simulink model "LLC_simscape3"  (R2022b)
settings: Solver=VariableStepAuto  StartTime=0.0  StopTime=0.1  MaxStep=1e-4  RelTol=1e-4
PreLoadFcn:
  | Rs_fet=1e8;  % FET snubber resistance (ohms)
  | Cs_fet=inf;  % FET snubber capacitance (ohms)
  | Vf=0.6;        % Diode forward voltage (V)
libraries: spsSeriesRLCBranchLib x10, spsVoltageMeasurementLib x7, spsCurrentMeasurementLib x5, spsControlledVoltageSourceLib x2, spsGroundLib x2, spsNonlinearInductorLib x2, spsACVoltageSourceLib x1, spspowerguiLib x1
settings Model: SimulationMode=accelerator  PauseTimes=0.001  Creator=Hyeongmeen Baik  LastModifiedBy=Hyeongmeen Baik
settings ModelReferenceCC: UpdateModelReferenceTargets=IfOutOfDate  EnableRefExpFcnMdlSchedulingChecks=on

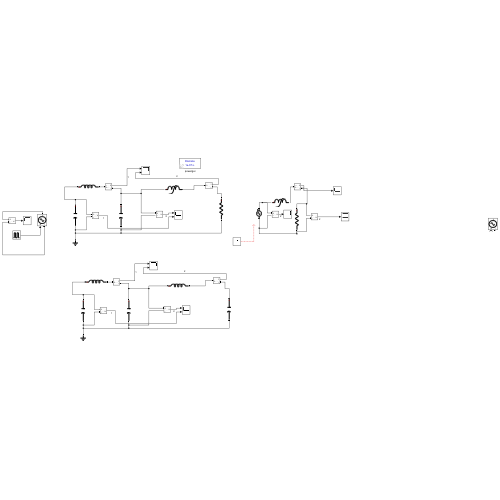
[thumbnail: Simulink's stored preview of the top-level diagram]
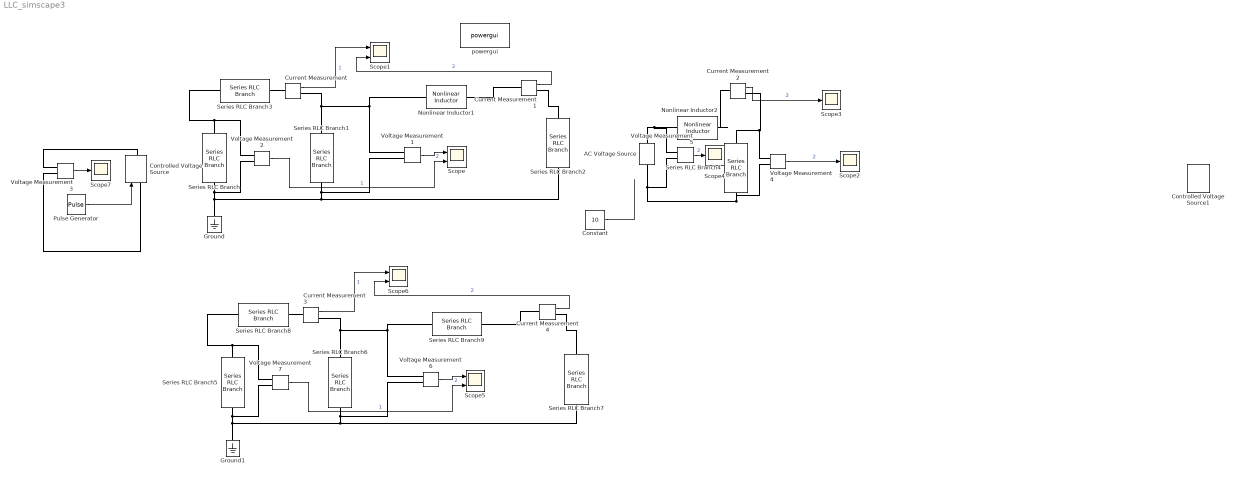
== system LLC_simscape3 ==
  AC Voltage Source : spsACVoltageSourceLib/AC Voltage Source  Amplitude=1500  Phase=0  Frequency=10  SampleTime=0  Measurements=None  BusType=swing  Pref=10e3  Qref=0  Qmin=-inf  Qmax=+inf
  Constant : Constant  Value=10
  Controlled Voltage Source : spsControlledVoltageSourceLib/Controlled Voltage Source  Initialize=on  Source_Type=AC  Amplitude=0  Phase=0  Frequency=0  Measurements=None
  Controlled Voltage Source1 : spsControlledVoltageSourceLib/Controlled Voltage Source  Initialize=on  Source_Type=AC  Amplitude=0  Phase=0  Frequency=0  Measurements=None
  Current Measurement{,1..4} (5 alike) : spsCurrentMeasurementLib/Current Measurement  PhasorSimulation=off  OutputType=Complex  PSBequivalent=0
  Ground : spsGroundLib/Ground  LConnTagsString=a
  Ground1 : spsGroundLib/Ground  LConnTagsString=a
  Nonlinear Inductor1 : spsNonlinearInductorLib/Nonlinear Inductor  DiscreteSolver=Backward Euler  VI=flux_current2  IFL=0  Measurements=Flux, Imag
      settings: LibrarySourceBlock=sps_lib/Passives/Nonlinear Inductor
  Nonlinear Inductor2 : spsNonlinearInductorLib/Nonlinear Inductor  DiscreteSolver=Backward Euler  VI=flux_current2  IFL=0  Measurements=Flux, Imag
      settings: LibrarySourceBlock=sps_lib/Passives/Nonlinear Inductor
  Pulse Generator : DiscretePulseGenerator  PulseType=Time based  Period=0.1  PulseWidth=5
  Scope{,1,5..6} (4 alike) : Scope  NumInputPorts=2
  Scope{2..4,7} (4 alike) : Scope
  Series RLC Branch : spsSeriesRLCBranchLib/Series RLC Branch  LConnTagsString=__new0  RConnTagsString=__new0  BranchType=C  Resistance=1  Inductance=1e-3  SetiL0=off  InitialCurrent=0  Capacitance=1e-3  Setx0=on  InitialVoltage=1500  Measurements=None
  Series RLC Branch1 : spsSeriesRLCBranchLib/Series RLC Branch  LConnTagsString=__new0  RConnTagsString=__new0  BranchType=C  Resistance=1  Inductance=1e-3  SetiL0=off  InitialCurrent=0  Capacitance=1e-3  Setx0=off  InitialVoltage=0  Measurements=None
  Series RLC Branch2 : spsSeriesRLCBranchLib/Series RLC Branch  LConnTagsString=__new0  RConnTagsString=__new0  BranchType=R  Resistance=1  Inductance=1e-3  SetiL0=off  InitialCurrent=0  Capacitance=1e-6  Setx0=off  InitialVoltage=0  Measurements=None
  Series RLC Branch3 : spsSeriesRLCBranchLib/Series RLC Branch  LConnTagsString=__new0  RConnTagsString=__new0  BranchType=L  Resistance=1  Inductance=1e-3  SetiL0=off  InitialCurrent=0  Capacitance=1e-6  Setx0=off  InitialVoltage=0  Measurements=None
  Series RLC Branch4 : spsSeriesRLCBranchLib/Series RLC Branch  LConnTagsString=__new0  RConnTagsString=__new0  BranchType=R  Resistance=1  Inductance=1e-3  SetiL0=off  InitialCurrent=0  Capacitance=1e-6  Setx0=off  InitialVoltage=0  Measurements=None
  Series RLC Branch5 : spsSeriesRLCBranchLib/Series RLC Branch  LConnTagsString=__new0  RConnTagsString=__new0  BranchType=C  Resistance=1  Inductance=1e-3  SetiL0=off  InitialCurrent=0  Capacitance=1e-3  Setx0=on  InitialVoltage=1500  Measurements=None
  Series RLC Branch6 : spsSeriesRLCBranchLib/Series RLC Branch  LConnTagsString=__new0  RConnTagsString=__new0  BranchType=C  Resistance=1  Inductance=1e-3  SetiL0=off  InitialCurrent=0  Capacitance=1e-3  Setx0=off  InitialVoltage=0  Measurements=None
  Series RLC Branch7 : spsSeriesRLCBranchLib/Series RLC Branch  LConnTagsString=__new0  RConnTagsString=__new0  BranchType=C  Resistance=1  Inductance=1e-3  SetiL0=off  InitialCurrent=0  Capacitance=1e-3  Setx0=off  InitialVoltage=0  Measurements=None
  Series RLC Branch8 : spsSeriesRLCBranchLib/Series RLC Branch  LConnTagsString=__new0  RConnTagsString=__new0  BranchType=L  Resistance=1  Inductance=1e-3  SetiL0=off  InitialCurrent=0  Capacitance=1e-6  Setx0=off  InitialVoltage=0  Measurements=None
  Series RLC Branch9 : spsSeriesRLCBranchLib/Series RLC Branch  LConnTagsString=__new0  RConnTagsString=__new0  BranchType=L  Resistance=1  Inductance=1e-1  SetiL0=off  InitialCurrent=0  Capacitance=1e-6  Setx0=off  InitialVoltage=0  Measurements=None
  Voltage Measurement{1..7} (7 alike) : spsVoltageMeasurementLib/Voltage Measurement  PhasorSimulation=off  OutputType=Complex  PSBequivalent=0
  powergui : spspowerguiLib/powergui  Priority=1  SimulationMode=Discrete  SampleTime=1e-7  frequency=60  Iterations=50  frequencyindice=0  Pbase=100e6  ErrMax=1e-4  UnitsV=kV  UnitsW=MW  buscounter=0  FunctionMessages=off  echomessages=off  EnableUseOfTLC=off  CurrentSourceSwitches=off  DisableSnubberDevices=off  DisableRonSwitches=off  DisableVfSwitches=off  DisplayEquations=off  AutomaticDiscreteSolvers=off  SolverType=Tustin/Backward Euler (TBE)  Interpol=off  ExternalGateDelay=off  methode=off  Ts=100  x0status=blocks  SPID=on  SwTol=0  HookPort=off  NonlinearTolerance=1e-4  nMaxIteration=100  ContinueOnMaxIteration=off  RestoreLinks=warning  ResistiveCurrentMeasurement=off  Frange=[0:2:500]  Ylog=off  Xlog=on  ShowGrid=off  save=off  variable=ZData  structure=0  ZoomFFT=off  StartTime=0.0  cycles=1  DisplayStyle=1  fundamental=60  FreqAxis=off  MaxFrequency=1000  frequencyindicesteady=1  RmsSteady=1  display=off
  wires:
  Pulse Generator/1 -> Controlled Voltage Source/1
  Voltage Measurement3/1 -> Scope7/1
  Voltage Measurement1/1 -> Scope/1  "2"
  Current Measurement/1 -> Scope1/1  "1"
  Current Measurement1/1 -> Scope1/2  "2"
  Voltage Measurement2/1 -> Scope/2  "1"
  Constant/1 -> ?
  Voltage Measurement4/1 -> Scope2/1  "2"
  Current Measurement2/1 -> Scope3/1  "2"
  Voltage Measurement5/1 -> Scope4/1  "2"
  Current Measurement4/1 -> Scope6/2  "2"
  Voltage Measurement7/1 -> Scope5/2  "1"
  Current Measurement3/1 -> Scope6/1  "1"
  Voltage Measurement6/1 -> Scope5/1  "2"
  connections:
  Voltage Measurement3/LConn1 -- Controlled Voltage Source/RConn1
  Voltage Measurement3/LConn2 -- Controlled Voltage Source/LConn1
  Ground/LConn1 -- Series RLC Branch2/RConn1 -- Voltage Measurement1/LConn2 -- Series RLC Branch1/RConn1 -- Voltage Measurement2/LConn2 -- Series RLC Branch/RConn1
  Series RLC Branch3/LConn1 -- Voltage Measurement2/LConn1 -- Series RLC Branch/LConn1
  Voltage Measurement1/LConn1 -- Nonlinear Inductor1/LConn1 -- Current Measurement/RConn1 -- Series RLC Branch1/LConn1
  Series RLC Branch3/RConn1 -- Current Measurement/LConn1
  Current Measurement1/RConn1 -- Series RLC Branch2/LConn1
  Nonlinear Inductor1/RConn1 -- Current Measurement1/LConn1
  Series RLC Branch4/LConn1 -- Current Measurement2/RConn1 -- Voltage Measurement4/LConn1
  Series RLC Branch4/RConn1 -- Voltage Measurement5/LConn2 -- AC Voltage Source/LConn1 -- Voltage Measurement4/LConn2
  AC Voltage Source/RConn1 -- Voltage Measurement5/LConn1 -- Nonlinear Inductor2/LConn1
  Nonlinear Inductor2/RConn1 -- Current Measurement2/LConn1
  Series RLC Branch6/LConn1 -- Series RLC Branch9/LConn1 -- Voltage Measurement6/LConn1 -- Current Measurement3/RConn1
  Series RLC Branch5/RConn1 -- Voltage Measurement7/LConn2 -- Series RLC Branch7/RConn1 -- Voltage Measurement6/LConn2 -- Series RLC Branch6/RConn1 -- Ground1/LConn1
  Series RLC Branch8/LConn1 -- Voltage Measurement7/LConn1 -- Series RLC Branch5/LConn1
  Current Measurement4/RConn1 -- Series RLC Branch7/LConn1
  Current Measurement4/LConn1 -- Series RLC Branch9/RConn1
  Series RLC Branch8/RConn1 -- Current Measurement3/LConn1
